simulink model "second_order_sim"  (R2023a)
settings: Solver=VariableStepAuto  StartTime=0.0  StopTime=10.0  RelTol=1e-3
values from neighbouring files (symbols this model uses):
  wn = 10    [SCRIPT_second_order.m]
  zeta = 1.5    [SCRIPT_second_order.m]
settings Model: Creator=mazen  LastModifiedBy=mazen

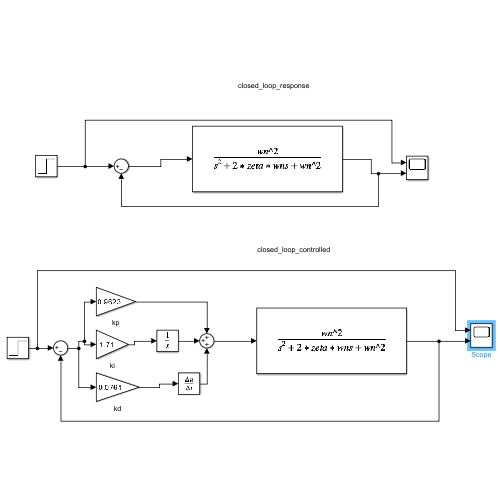
[thumbnail: Simulink's stored preview of the top-level diagram]
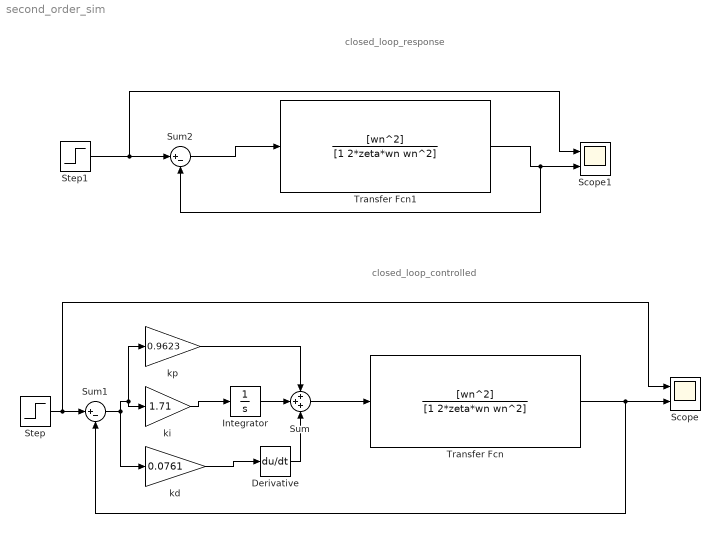
== system second_order_sim ==
  note: closed_loop_controlled
  note: closed_loop_response
  Derivative : Derivative
  Integrator : Integrator
  Scope : Scope  NumInputPorts=2
  Scope1 : Scope  NumInputPorts=2
  Step : Step  SampleTime=0
  Step1 : Step  SampleTime=0
  Sum : Sum  Inputs=+++
  Sum1 : Sum  Inputs=|+-
  Sum2 : Sum  Inputs=|+-
  Transfer Fcn : TransferFcn  Numerator=[wn^2]  Denominator=[1 2*zeta*wn wn^2]
  Transfer Fcn1 : TransferFcn  Numerator=[wn^2]  Denominator=[1 2*zeta*wn wn^2]
  kd : Gain  Gain=0.0761
  ki : Gain  Gain=1.71
  kp : Gain  Gain=0.9623
  wires:
  ki/1 -> Integrator/1
  kd/1 -> Derivative/1
  Integrator/1 -> Sum/2
  kp/1 -> Sum/1
  Derivative/1 -> Sum/3
  Sum/1 -> Transfer Fcn/1
  Step/1 -> Scope/1, Sum1/1
  Sum1/1 -> kp/1, ki/1, kd/1
  Transfer Fcn/1 -> Sum1/2, Scope/2
  Transfer Fcn1/1 -> Sum2/2, Scope1/2
  Sum2/1 -> Transfer Fcn1/1
  Step1/1 -> Scope1/1, Sum2/1
